simulink model "Factorial_Matlab_fn__For_Loop"  (R2018a)
settings: Solver=VariableStepAuto  StartTime=0.0  StopTime=10.0  RelTol=1e-3
settings Model: Creator=Moataz  LastModifiedBy=Moataz

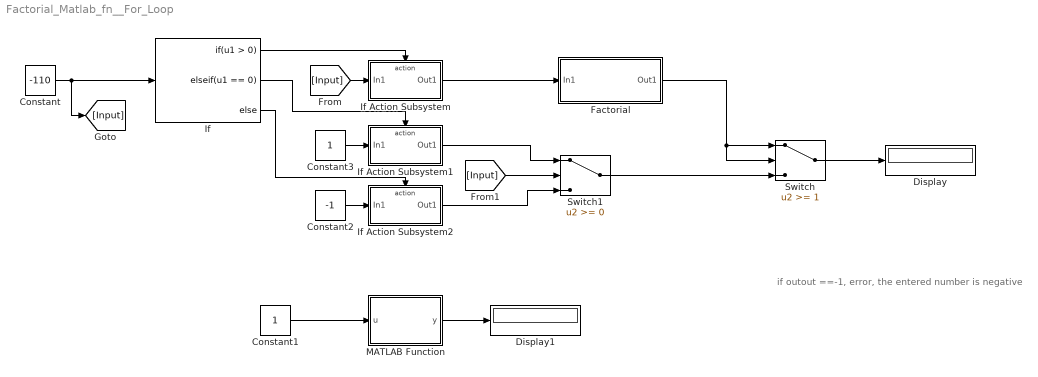
== system Factorial_Matlab_fn__For_Loop ==
  note: if outout ==-1, error, the entered number is negative
  Constant : Constant  Value=-110  OutDataTypeStr=int32
  Constant1 : Constant
  Constant2 : Constant  Value=-1
  Constant3 : Constant
  Display : Display
  Display1 : Display
  "Factorial " : Subsystem  TreatAsAtomicUnit=on
  If : If  ElseIfExpressions=u1 == 0
  If Action Subsystem : Subsystem  TreatAsAtomicUnit=on
  If Action Subsystem1 : Subsystem  TreatAsAtomicUnit=on
  If Action Subsystem2 : Subsystem  TreatAsAtomicUnit=on
  MATLAB Function : MATLAB Function  TreatAsAtomicUnit=on
  Switch : Switch  Threshold=1
  Switch1 : Switch
  wires:
  Constant1/1 -> MATLAB Function/1(u)
  MATLAB Function/1(y) -> Display1/1
  Constant/1 -> [Input], If/1
  If Action Subsystem/1(Out1) -> "Factorial "/1(In1)
  If/1 -> If Action Subsystem/Action
  If/2 -> If Action Subsystem1/Action
  Constant3/1 -> If Action Subsystem1/1(In1)
  If/3 -> If Action Subsystem2/Action
  Constant2/1 -> If Action Subsystem2/1(In1)
  [Input] -> If Action Subsystem/1(In1)
  Switch/1 -> Display/1
  "Factorial "/1(Out1) -> Switch/2, Switch/1
  Switch1/1 -> Switch/3
  If Action Subsystem1/1(Out1) -> Switch1/1
  If Action Subsystem2/1(Out1) -> Switch1/3
  [Input] -> Switch1/2

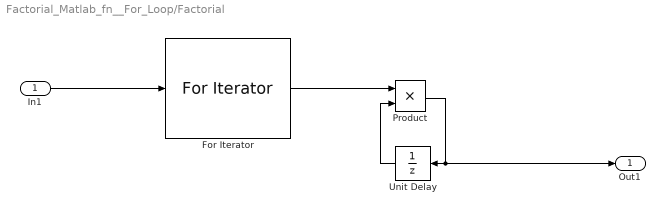
== system Factorial_Matlab_fn__For_Loop/Factorial  ==
  In1 : Inport  OutDataTypeStr=int32
  For Iterator : ForIterator  ResetStates=reset  IterationSource=external
  Product : Product  OutDataTypeStr=int32
  Unit Delay : UnitDelay  InitialCondition=1  SampleTime=-1
  Out1 : Outport
  wires:
  For Iterator/1 -> Product/1
  Unit Delay/1 -> Product/2
  In1/1 -> For Iterator/1
  Product/1 -> Unit Delay/1, Out1/1

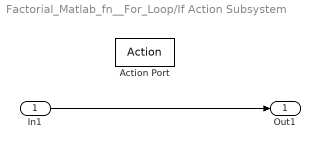
== system Factorial_Matlab_fn__For_Loop/If Action Subsystem ==
  In1 : Inport  OutDataTypeStr=int32
  Action Port : ActionPort  ActionType=then
  Out1 : Outport  OutDataTypeStr=int32
  wires:
  In1/1 -> Out1/1

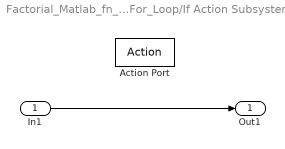
== system Factorial_Matlab_fn__For_Loop/If Action Subsystem1 ==
  In1 : Inport
  Action Port : ActionPort  ActionType=elseif
  Out1 : Outport
  wires:
  In1/1 -> Out1/1

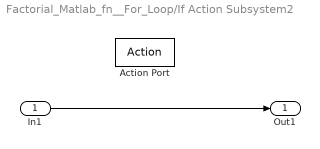
== system Factorial_Matlab_fn__For_Loop/If Action Subsystem2 ==
  In1 : Inport
  Action Port : ActionPort  ActionType=else
  Out1 : Outport
  wires:
  In1/1 -> Out1/1

== matlab function Factorial_Matlab_fn__For_Loop/MATLAB Function ==
  data: u input; y output
function y = fcn(u)
y=1;
if u<0
    y=-1


else
    for i=u:-1:1
        y=y*i
    end
end
